simulink model "ElectronicThrottleController"  (R2022b)
settings: Solver=VariableStepAuto  StartTime=0.0  StopTime=10.0  RelTol=1e-3
undefined symbols (not defined in the file or in its folder): TPS_Modes
settings Model: Creator=ahmed  LastModifiedBy=ahmed

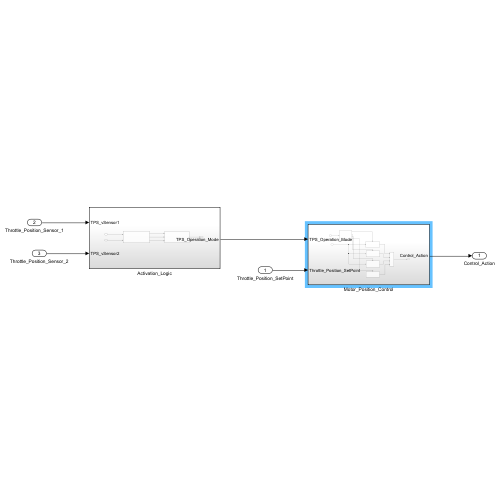
[thumbnail: Simulink's stored preview of the top-level diagram]
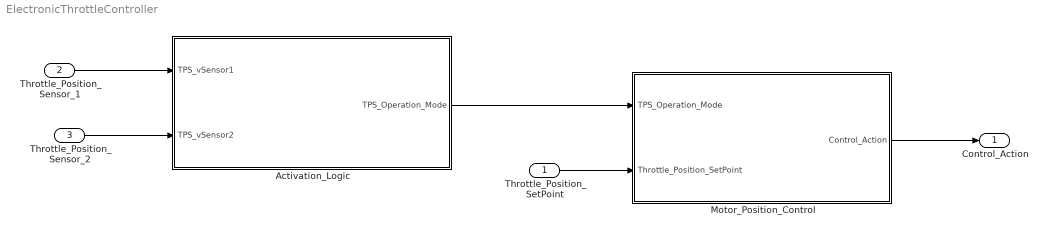
== system ElectronicThrottleController ==
  Throttle_Position_SetPoint : Inport
  Throttle_Position_Sensor_1 : Inport  Port=2
  Throttle_Position_Sensor_2 : Inport  Port=3
  Activation_Logic : Subsystem
  Motor_Position_Control : Subsystem
  Control_Action : Outport
  wires:
  Throttle_Position_Sensor_1/1 -> Activation_Logic/1(TPS_vSensor1)
  Throttle_Position_Sensor_2/1 -> Activation_Logic/2(TPS_vSensor2)
  Activation_Logic/1(TPS_Operation_Mode) -> Motor_Position_Control/1(TPS_Operation_Mode)
  Throttle_Position_SetPoint/1 -> Motor_Position_Control/2(Throttle_Position_SetPoint)
  Motor_Position_Control/1(Control_Action) -> Control_Action/1

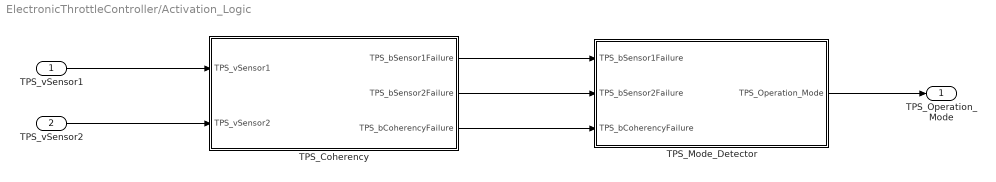
== system ElectronicThrottleController/Activation_Logic ==
  TPS_vSensor1 : Inport
  TPS_vSensor2 : Inport  Port=2
  TPS_Coherency : Subsystem
  TPS_Mode_Detector : Subsystem
  TPS_Operation_Mode : Outport  OutDataTypeStr=Enum: TPS_Modes
  wires:
  TPS_vSensor2/1 -> TPS_Coherency/2(TPS_vSensor2)
  TPS_Coherency/3(TPS_bCoherencyFailure) -> TPS_Mode_Detector/3(TPS_bCoherencyFailure)
  TPS_Mode_Detector/1(TPS_Operation_Mode) -> TPS_Operation_Mode/1
  TPS_Coherency/1(TPS_bSensor1Failure) -> TPS_Mode_Detector/1(TPS_bSensor1Failure)
  TPS_vSensor1/1 -> TPS_Coherency/1(TPS_vSensor1)
  TPS_Coherency/2(TPS_bSensor2Failure) -> TPS_Mode_Detector/2(TPS_bSensor2Failure)

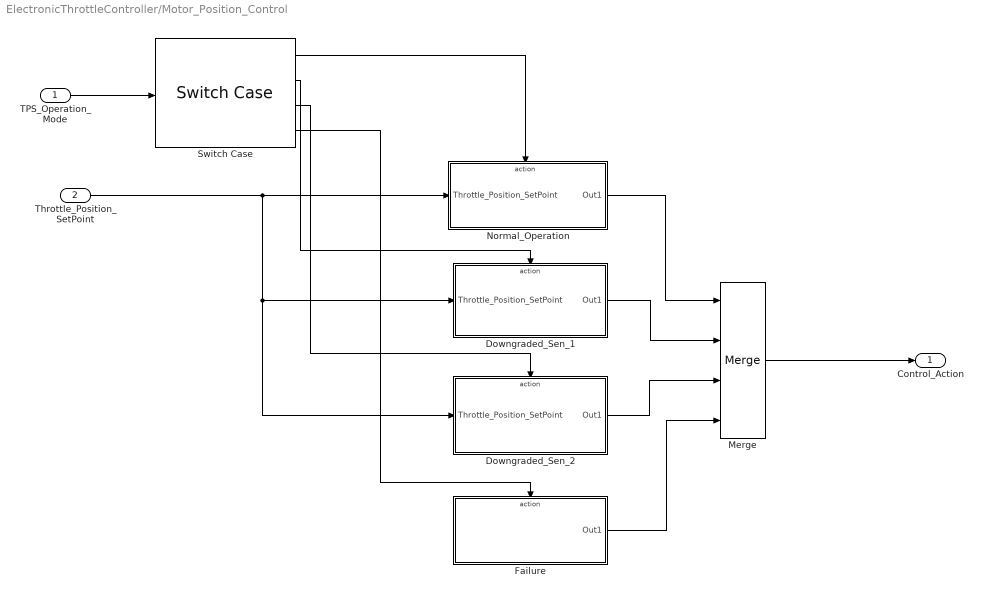
== system ElectronicThrottleController/Motor_Position_Control ==
  TPS_Operation_Mode : Inport  OutDataTypeStr=Enum: TPS_Modes
  Throttle_Position_SetPoint : Inport  Port=2
  Downgraded_Sen_1 : Subsystem  TreatAsAtomicUnit=on
  Downgraded_Sen_2 : Subsystem  TreatAsAtomicUnit=on
  Failure : Subsystem  TreatAsAtomicUnit=on
  Merge : Merge  Inputs=4
  Normal_Operation : Subsystem  TreatAsAtomicUnit=on
  Switch Case : SwitchCase  CaseConditions={TPS_Modes.Normal,TPS_Modes.Downgraded_Sen_1,TPS_Modes.Downgraded_Sen_2,TPS_Modes.Failure_Mode}  ShowDefaultCase=off
  Control_Action : Outport
  wires:
  Switch Case/4 -> Failure/Action
  Merge/1 -> Control_Action/1
  Throttle_Position_SetPoint/1 -> Downgraded_Sen_2/1(Throttle_Position_SetPoint), Downgraded_Sen_1/1(Throttle_Position_SetPoint), Normal_Operation/1(Throttle_Position_SetPoint)
  Normal_Operation/1(Out1) -> Merge/1
  Failure/1(Out1) -> Merge/4
  Downgraded_Sen_1/1(Out1) -> Merge/2
  Downgraded_Sen_2/1(Out1) -> Merge/3
  Switch Case/1 -> Normal_Operation/Action
  Switch Case/2 -> Downgraded_Sen_1/Action
  Switch Case/3 -> Downgraded_Sen_2/Action
  TPS_Operation_Mode/1 -> Switch Case/1

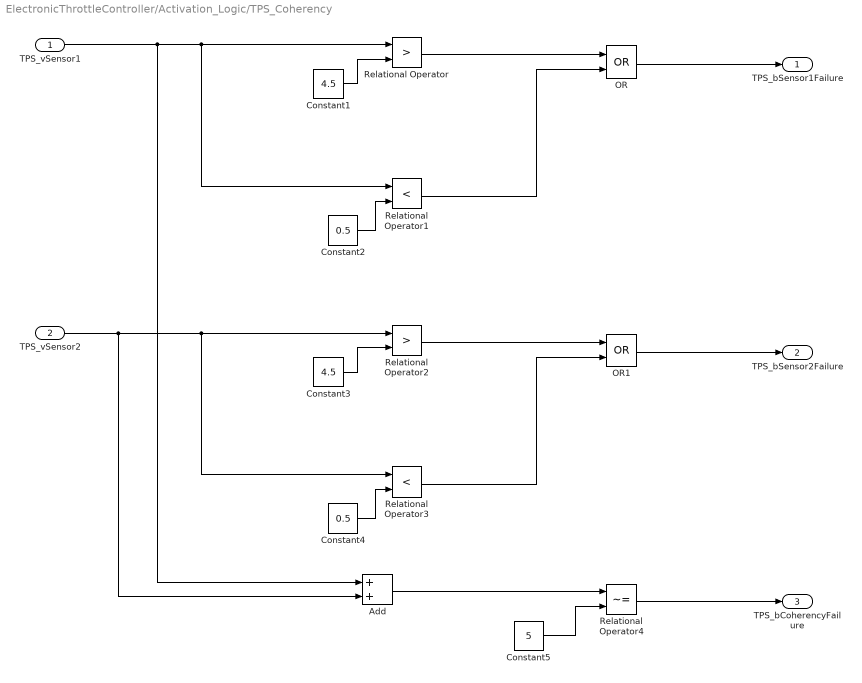
== system ElectronicThrottleController/Activation_Logic/TPS_Coherency ==
  TPS_vSensor1 : Inport  OutDataTypeStr=single
  TPS_vSensor2 : Inport  Port=2  OutDataTypeStr=single
  Add : Sum
  Constant1 : Constant  Value=4.5
  Constant2 : Constant  Value=0.5
  Constant3 : Constant  Value=4.5
  Constant4 : Constant  Value=0.5
  Constant5 : Constant  Value=5
  OR : Logic  Operator=OR  AllPortsSameDT=off  OutDataTypeStr=boolean
  OR1 : Logic  Operator=OR  AllPortsSameDT=off  OutDataTypeStr=boolean
  Relational Operator : RelationalOperator  Operator=>  OutDataTypeStr=boolean  RndMeth=Simplest  InputSameDT=off
  Relational Operator1 : RelationalOperator  Operator=<  OutDataTypeStr=boolean  RndMeth=Simplest  InputSameDT=off
  Relational Operator2 : RelationalOperator  Operator=>  OutDataTypeStr=boolean  RndMeth=Simplest  InputSameDT=off
  Relational Operator3 : RelationalOperator  Operator=<  OutDataTypeStr=boolean  RndMeth=Simplest  InputSameDT=off
  Relational Operator4 : RelationalOperator  Operator=~=  OutDataTypeStr=boolean  RndMeth=Simplest  InputSameDT=off
  TPS_bSensor1Failure : Outport  OutDataTypeStr=boolean
  TPS_bSensor2Failure : Outport  Port=2  OutDataTypeStr=boolean
  TPS_bCoherencyFailure : Outport  Port=3  OutDataTypeStr=boolean
  wires:
  Constant2/1 -> Relational Operator1/2
  Relational Operator3/1 -> OR1/2
  Relational Operator/1 -> OR/1
  TPS_vSensor2/1 -> Relational Operator3/1, Relational Operator2/1, Add/2
  Constant4/1 -> Relational Operator3/2
  Constant1/1 -> Relational Operator/2
  Relational Operator2/1 -> OR1/1
  OR1/1 -> TPS_bSensor2Failure/1
  TPS_vSensor1/1 -> Relational Operator1/1, Relational Operator/1, Add/1
  Relational Operator4/1 -> TPS_bCoherencyFailure/1
  Constant5/1 -> Relational Operator4/2
  Add/1 -> Relational Operator4/1
  Constant3/1 -> Relational Operator2/2
  Relational Operator1/1 -> OR/2
  OR/1 -> TPS_bSensor1Failure/1

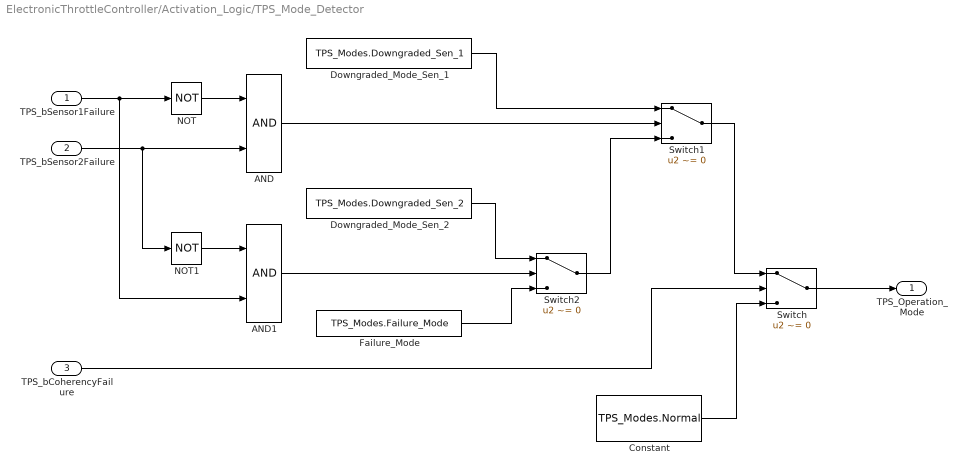
== system ElectronicThrottleController/Activation_Logic/TPS_Mode_Detector ==
  TPS_bSensor1Failure : Inport  OutDataTypeStr=boolean
  TPS_bSensor2Failure : Inport  Port=2  OutDataTypeStr=boolean
  TPS_bCoherencyFailure : Inport  Port=3  OutDataTypeStr=boolean
  AND : Logic  AllPortsSameDT=off  OutDataTypeStr=boolean
  AND1 : Logic  AllPortsSameDT=off  OutDataTypeStr=boolean
  Constant : Constant  Value=TPS_Modes.Normal
  Downgraded_Mode_Sen_1 : Constant  Value=TPS_Modes.Downgraded_Sen_1
  Downgraded_Mode_Sen_2 : Constant  Value=TPS_Modes.Downgraded_Sen_2
  Failure_Mode : Constant  Value=TPS_Modes.Failure_Mode
  NOT : Logic  Operator=NOT  AllPortsSameDT=off  OutDataTypeStr=boolean
  NOT1 : Logic  Operator=NOT  AllPortsSameDT=off  OutDataTypeStr=boolean
  Switch : Switch  Criteria=u2 ~= 0  SaturateOnIntegerOverflow=off  InputSameDT=off
  Switch1 : Switch  Criteria=u2 ~= 0  SaturateOnIntegerOverflow=off  InputSameDT=off
  Switch2 : Switch  Criteria=u2 ~= 0  SaturateOnIntegerOverflow=off  InputSameDT=off
  TPS_Operation_Mode : Outport  OutDataTypeStr=Enum: TPS_Modes
  wires:
  TPS_bCoherencyFailure/1 -> Switch/2
  Constant/1 -> Switch/3
  TPS_bSensor1Failure/1 -> NOT/1, AND1/2
  NOT/1 -> AND/1
  TPS_bSensor2Failure/1 -> AND/2, NOT1/1
  AND/1 -> Switch1/2
  Downgraded_Mode_Sen_1/1 -> Switch1/1
  NOT1/1 -> AND1/1
  Downgraded_Mode_Sen_2/1 -> Switch2/1
  AND1/1 -> Switch2/2
  Failure_Mode/1 -> Switch2/3
  Switch2/1 -> Switch1/3
  Switch1/1 -> Switch/1
  Switch/1 -> TPS_Operation_Mode/1

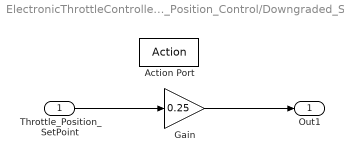
== system ElectronicThrottleController/Motor_Position_Control/Downgraded_Sen_1 ==
  Throttle_Position_SetPoint : Inport
  Action Port : ActionPort  ActionPortLabel=case [ Downgraded_Sen_1 ]:
  Gain : Gain  Gain=0.25
  Out1 : Outport
  wires:
  Throttle_Position_SetPoint/1 -> Gain/1
  Gain/1 -> Out1/1

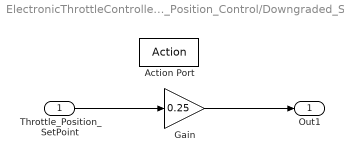
== system ElectronicThrottleController/Motor_Position_Control/Downgraded_Sen_2 ==
  Throttle_Position_SetPoint : Inport
  Action Port : ActionPort  ActionPortLabel=case [ Downgraded_Sen_2 ]:
  Gain : Gain  Gain=0.25
  Out1 : Outport
  wires:
  Throttle_Position_SetPoint/1 -> Gain/1
  Gain/1 -> Out1/1

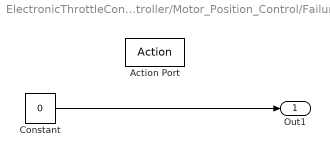
== system ElectronicThrottleController/Motor_Position_Control/Failure ==
  Action Port : ActionPort  ActionPortLabel=case [ Failure_Mode ]:
  Constant : Constant  Value=0
  Out1 : Outport
  wires:
  Constant/1 -> Out1/1

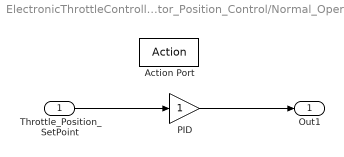
== system ElectronicThrottleController/Motor_Position_Control/Normal_Operation ==
  Throttle_Position_SetPoint : Inport
  Action Port : ActionPort  ActionPortLabel=case [ Normal ]:
  "PID " : Gain
  Out1 : Outport
  wires:
  Throttle_Position_SetPoint/1 -> "PID "/1
  "PID "/1 -> Out1/1
